simulink model "dual_mass"  (R2023a)
settings: Solver=VariableStepAuto  StartTime=0.0  StopTime=10  RelTol=1e-3
values from neighbouring files (symbols this model uses):
  Ad = SYSd.A    [dual_param.m]
  Bd = SYSd.B    [dual_param.m]
  Cd = SYSd.C    [dual_param.m]
  Dd = SYSd.D    [dual_param.m]
  Nx = [1 0 1 0; 0 0 0 0]    [dual_param.m]
  Ts = 1E-3    (= 0.001)    [dual_param.m]
undefined symbols (not defined in the file or in its folder): K
settings Model: Creator=Admin  LastModifiedBy=Admin
settings ModelReferenceCC: EnableRefExpFcnMdlSchedulingChecks=on

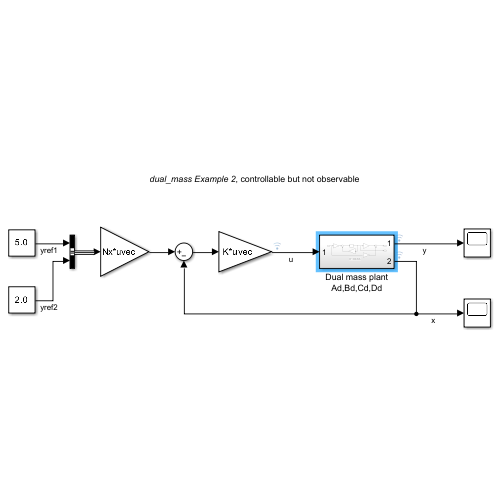
[thumbnail: Simulink's stored preview of the top-level diagram]
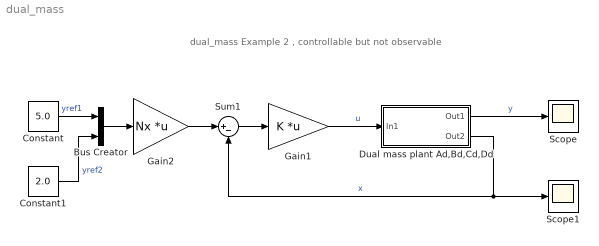
== system dual_mass ==
  note: dual_mass Example 2 , controllable but not observable
  Bus Creator : BusCreator  Inputs=2
  Constant : Constant  Value=5.0  SampleTime=Ts
  Constant1 : Constant  Value=2.0  SampleTime=Ts
  Dual mass plant Ad,Bd,Cd,Dd : Subsystem
  Gain1 : Gain  Gain=K  Multiplication=Matrix(K*u) (u vector)
  Gain2 : Gain  Gain=Nx  Multiplication=Matrix(K*u) (u vector)
  Scope : Scope
  Scope1 : Scope
  Sum1 : Sum  Inputs=|+-
  wires:
  Dual mass plant Ad,Bd,Cd,Dd/1(Out1) -> Scope/1  "y"
  Dual mass plant Ad,Bd,Cd,Dd/2(Out2) -> Sum1/2, Scope1/1  "x"
  Gain1/1 -> Dual mass plant Ad,Bd,Cd,Dd/1(In1)  "u"
  Sum1/1 -> Gain1/1
  Constant/1 -> Bus Creator/1  "yref1"
  Bus Creator/1 -> Gain2/1
  Gain2/1 -> Sum1/1
  Constant1/1 -> Bus Creator/2  "yref2"

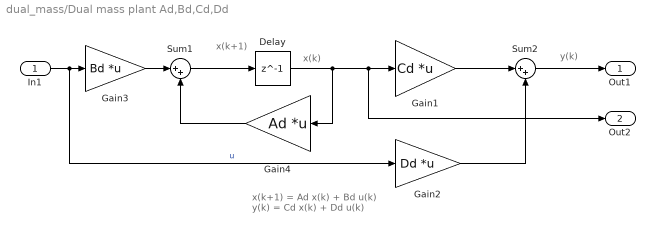
== system dual_mass/Dual mass plant Ad,Bd,Cd,Dd ==
  note: x(k)
  note: x(k+1) = Ad x(k) + Bd u(k)
      | y(k) = Cd x(k) + Dd u(k)
  note: x(k+1)
  note: y(k)
  In1 : Inport
  Delay : Delay  DelayLength=1
  Gain1 : Gain  Gain=Cd  Multiplication=Matrix(K*u) (u vector)
  Gain2 : Gain  Gain=Dd  Multiplication=Matrix(K*u) (u vector)
  Gain3 : Gain  Gain=Bd  Multiplication=Matrix(K*u) (u vector)
  Gain4 : Gain  Gain=Ad  Multiplication=Matrix(K*u) (u vector)
  Sum1 : Sum  Inputs=|++
  Sum2 : Sum  Inputs=|++
  Out1 : Outport
  Out2 : Outport  Port=2
  wires:
  In1/1 -> Gain2/1, Gain3/1  "u"
  Sum1/1 -> Delay/1
  Delay/1 -> Gain4/1, Out2/1, Gain1/1
  Gain3/1 -> Sum1/1
  Gain4/1 -> Sum1/2
  Sum2/1 -> Out1/1
  Gain1/1 -> Sum2/1
  Gain2/1 -> Sum2/2
